simulink model "tema2_mdl1"  (R2019a)
settings: Solver=VariableStepAuto  StartTime=0.0  StopTime=400  RelTol=1e-3
values from neighbouring files (symbols this model uses):
  r = 2 * ystar    [tema2.m]
  sys = ss(S.a, S.b, S.c, S.d)    [tema2.m]
  ustar = zeros(10,1)    [tema1.m]
undefined symbols (not defined in the file or in its folder): xstar, ystar
settings Model: Creator=cynthia  LastModifiedBy=cynthia

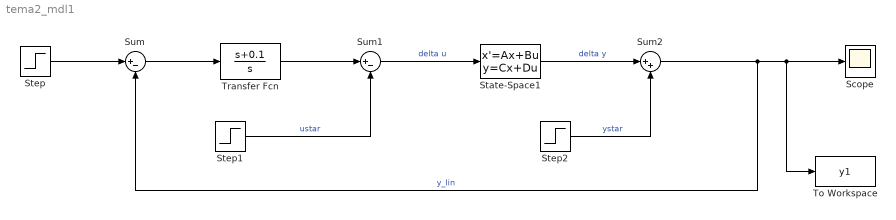
== system tema2_mdl1 ==
  Scope : Scope
  State-Space1 : StateSpace  A=sys.A  B=sys.B  C=sys.C  D=sys.D  InitialCondition=[0;0;0;0] - xstar
  Step : Step  Time=0  After=r  SampleTime=0
  Step1 : Step  Time=0  After=ustar  SampleTime=0
  Step2 : Step  Time=0  After=ystar  SampleTime=0
  Sum : Sum  Inputs=|+-
  Sum1 : Sum  Inputs=|+-
  Sum2 : Sum  Inputs=|++
  To Workspace : ToWorkspace  VariableName=y1  SaveFormat=Timeseries  SampleTime=-1
  Transfer Fcn : TransferFcn  Numerator=[1 0.1]  Denominator=[1 0 ]
  wires:
  State-Space1/1 -> Sum2/1  "delta y"
  Step1/1 -> Sum1/2  "ustar"
  Sum2/1 -> Sum/2, To Workspace/1, Scope/1  "y_lin"
  Sum1/1 -> State-Space1/1  "delta u"
  Step2/1 -> Sum2/2  "ystar"
  Transfer Fcn/1 -> Sum1/1
  Sum/1 -> Transfer Fcn/1
  Step/1 -> Sum/1
